simulink model "simlink_tp"  (R2023b)
settings: Solver=VariableStepAuto  StartTime=0.0  StopTime=10.0  RelTol=1e-3
libraries: dspsrcs4 x3
settings Model: Creator=rusha  LastModifiedBy=rusha

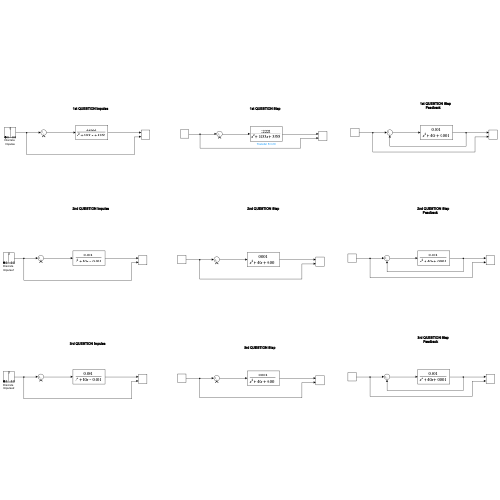
[thumbnail: Simulink's stored preview of the top-level diagram]
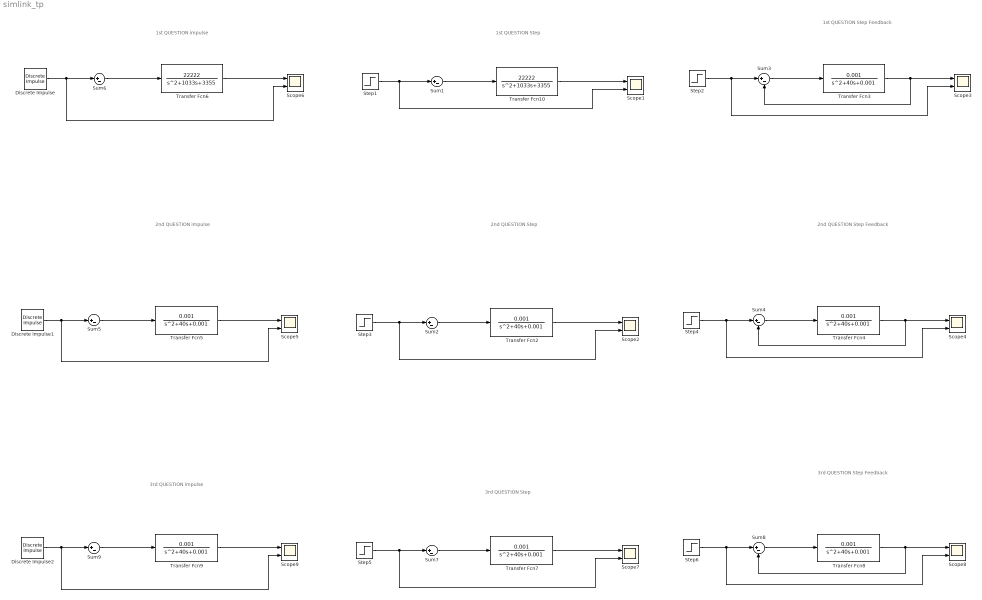
== system simlink_tp ==
  note: 1st QUESTION impulse
  note: 1st QUESTION Step
  note: 1st QUESTION Step Feedback
  note: 2nd QUESTION impulse
  note: 2nd QUESTION Step
  note: 2nd QUESTION Step Feedback
  note: 3rd QUESTION impulse
  note: 3rd QUESTION Step
  note: 3rd QUESTION Step Feedback
  Discrete Impulse : dspsrcs4/Discrete  Impulse  Delay=0  SampleTime=1  FrameSample=1  OutputFrames=off  dataType=double  isSigned=on  wordLen=16  udDataType=sfix(16)  fracBitsMode=Best precision  numFracBits=15  OutDataTypeStr=double  LastOutDataTypeStr=double
  Discrete Impulse1 : dspsrcs4/Discrete  Impulse  Delay=0  SampleTime=1  FrameSample=1  OutputFrames=off  dataType=double  isSigned=on  wordLen=16  udDataType=sfix(16)  fracBitsMode=Best precision  numFracBits=15  OutDataTypeStr=double  LastOutDataTypeStr=double
  Discrete Impulse2 : dspsrcs4/Discrete  Impulse  Delay=0  SampleTime=1  FrameSample=1  OutputFrames=off  dataType=double  isSigned=on  wordLen=16  udDataType=sfix(16)  fracBitsMode=Best precision  numFracBits=15  OutDataTypeStr=double  LastOutDataTypeStr=double
  Scope{1..9} (9 alike) : Scope  NumInputPorts=2
  Step{1..6} (6 alike) : Step  SampleTime=0
  Sum{1..9} (9 alike) : Sum  Inputs=|+-
  Transfer Fcn10 : TransferFcn  Numerator=[22222]  Denominator=[1 1033 3355]
  Transfer Fcn{2..5,7..9} (7 alike) : TransferFcn  Numerator=[0.001]  Denominator=[1 40 0.001]
  Transfer Fcn6 : TransferFcn  Numerator=[22222]  Denominator=[1 1033 3355]
  wires:
  Transfer Fcn6/1 -> Scope6/1
  Sum6/1 -> Transfer Fcn6/1
  Discrete Impulse/1 -> Scope6/2, Sum6/1
  Step1/1 -> Scope1/2, Sum1/1
  Sum1/1 -> Transfer Fcn10/1
  Transfer Fcn10/1 -> Scope1/1
  Transfer Fcn3/1 -> Sum3/2, Scope3/1
  Step2/1 -> Scope3/2, Sum3/1
  Sum3/1 -> Transfer Fcn3/1
  Sum2/1 -> Transfer Fcn2/1
  Step3/1 -> Scope2/2, Sum2/1
  Discrete Impulse1/1 -> Scope5/2, Sum5/1
  Step4/1 -> Scope4/2, Sum4/1
  Transfer Fcn4/1 -> Sum4/2, Scope4/1
  Sum4/1 -> Transfer Fcn4/1
  Transfer Fcn2/1 -> Scope2/1
  Transfer Fcn5/1 -> Scope5/1
  Sum5/1 -> Transfer Fcn5/1
  Sum7/1 -> Transfer Fcn7/1
  Step5/1 -> Scope7/2, Sum7/1
  Discrete Impulse2/1 -> Scope9/2, Sum9/1
  Step6/1 -> Scope8/2, Sum8/1
  Transfer Fcn8/1 -> Sum8/2, Scope8/1
  Sum8/1 -> Transfer Fcn8/1
  Transfer Fcn7/1 -> Scope7/1
  Transfer Fcn9/1 -> Scope9/1
  Sum9/1 -> Transfer Fcn9/1
